simulink model "SimDraft2"  (R2024a)
settings: Solver=VariableStepAuto  StartTime=0.0  StopTime=2  RelTol=1e-3
model workspace (MAT data in the model file):
  CanaryAmplitude = 0
  CanaryCarrierFrequency = 20000
  CanaryDataRate = 100
  DataAmplitude = 1
  SampleRate = 44100
undefined symbols (not defined in the file or in its folder): magnitude
libraries: dspfdesign x3, audiosources x2, commseqgen3 x2, commchan3 x1, commanapbnd3 x1, phasedenvlib x1, commsync2 x1
settings Model: Creator=calum  LastModifiedBy=calum

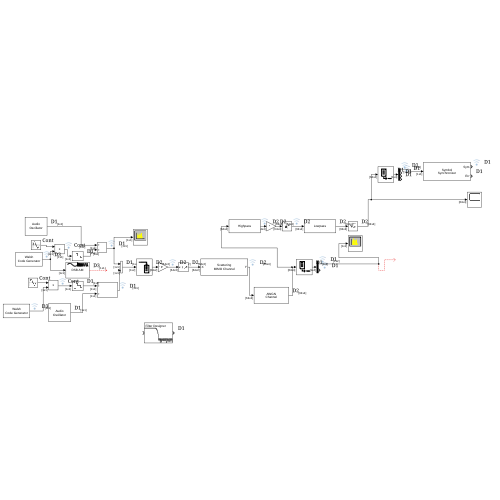
[thumbnail: Simulink's stored preview of the top-level diagram]
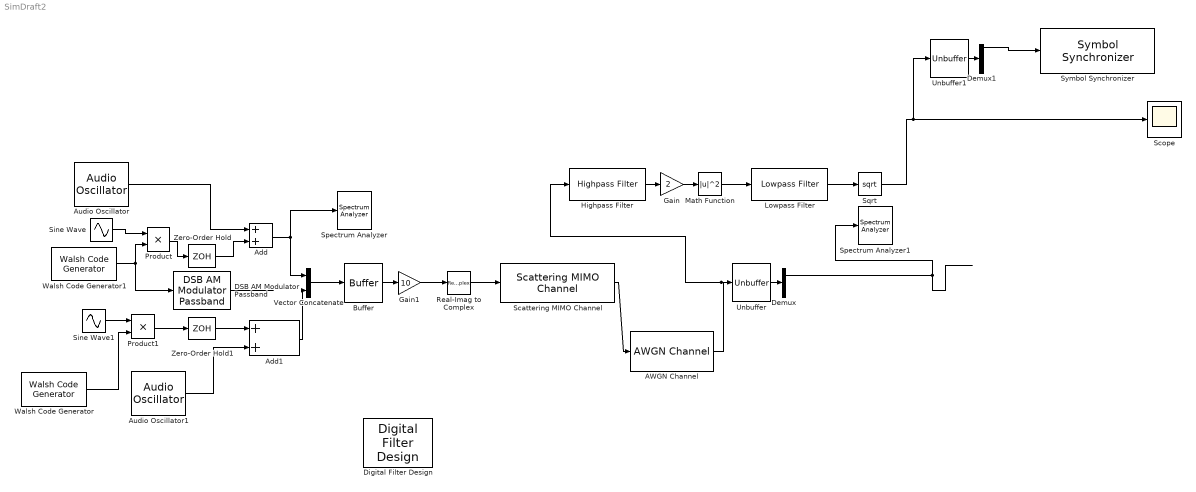
== system SimDraft2 ==
  AWGN Channel : commchan3/AWGN Channel  LegacyMode=off  NoiseMethod="Signal to noise ratio  (SNR)"  noiseMode="Signal to noise ratio  (SNR)"  EbNo=10  EsNo=10  SNR=70  BitsPerSymbol=1  SignalPower=1  SamplesPerSymbol=1  SymbolPeriod=1  VarianceSource=Parameter  Variance=1  RandomStream=Global stream  Seed=67  SimulateUsing=Code generation
  Add : Sum
  Add1 : Sum
  Audio Oscillator : audiosources/Audio Oscillator  FrequencyPort=off  Frequency=200  AmplitudePort=off  Amplitude=DataAmplitude  DCOffsetPort=off  DCOffset=0  PhaseOffset=0  WidthPort=off  Width=1  DutyCyclePort=off  DutyCycle=0.5  SampsPerFrame=1  Fs=SampleRate  OutputDataType=double  SimulateUsing=Code generation
      settings: SignalType=sine
  Audio Oscillator1 : audiosources/Audio Oscillator  FrequencyPort=off  Frequency=400  AmplitudePort=off  Amplitude=DataAmplitude  DCOffsetPort=off  DCOffset=0  PhaseOffset=0  WidthPort=off  Width=1  DutyCyclePort=off  DutyCycle=0.5  SampsPerFrame=1  Fs=SampleRate  OutputDataType=double  SimulateUsing=Code generation
      settings: SignalType=sine
  Buffer : Buffer  OutputFrames=off
  DSB AM Modulator Passband : commanapbnd3/DSB AM Modulator Passband  Fc=CanaryCarrierFrequency  Ph=0  Offset=1
  Demux : Demux  Outputs=2
  Demux1 : Demux
  Digital Filter Design : dspfdesign/Digital Filter Design  mwdsp_browser_bugfix_var=off
  Gain : Gain  Gain=2
  Gain1 : Gain  Gain=10
  Highpass Filter : dspfdesign/Highpass Filter  FilterType=FIR  DesignForMinimumOrder=on  FilterOrder=50  StopbandFrequency=CanaryCarrierFrequency-10*CanaryDataRate  PassbandFrequency=CanaryCarrierFrequency-4*CanaryDataRate  StopbandAttenuation=80  PassbandRipple=0.1  SampleRateMode=Specify on dialog  SampleRate=44100  SimulateUsing=Code generation  roundingMode=Floor  coeffsDataTypeStr=fixdt(1,16)
  Lowpass Filter : dspfdesign/Lowpass Filter  FilterType=FIR  DesignForMinimumOrder=on  FilterOrder=50  PassbandFrequency=CanaryDataRate  StopbandFrequency=CanaryDataRate*4  PassbandRipple=0.1  StopbandAttenuation=80  SampleRateMode=Specify on dialog  SampleRate=44100  SimulateUsing=Code generation  roundingMode=Floor  coeffsDataTypeStr=fixdt(1,16)
  Math Function : Math  Operator=magnitude^2
  Product : Product
  Product1 : Product
  Real-Imag to Complex : RealImagToComplex  Input=Real  ConstantPart=1E-3
  Scattering MIMO Channel : phasedenvlib/Scattering MIMO Channel  PropagationSpeed=300  CarrierFrequency=1  Polarization=None  SpecifyAtmosphere=off  Temperature=15  DryAirPressure=101325  WaterVapourDensity=7.5  LiquidWaterDensity=0  RainRate=0  SampleRateFromInputCheckbox=on  SampleRate=1e6  SimulateDirectPath=off  MaximumDelaySource=Property  MaximumDelay=2  ChannelResponseOutputPort=off  SimulateUsing=Code generation  TransmitArray=phased.ULA(Element=phased.OmnidirectionalMicrophoneElement(BackBaffled=false),ElementSpacing=20)  ReceiveArray=phased.ULA(Element=phased.OmnidirectionalMicrophoneElement(BackBaffled=false),ElementSpacing=10,NumElements=4)  TransmitArrayMotionSource=Property  TransmitArrayPosition=[ 0; 0; 0 ]  TransmitArrayOrientationAxes=eye( 3 )  ReceiveArrayMotionSource=Property  ReceiveArrayPosition=[ 1; 0; 0 ]  ReceiveArrayOrientationAxes=eye( 3 )  ScattererSpecificationSource=Property  NumScatterers=0  ScattererPositionBoundary=[ 0, 1000 ]  ScattererPosition=[ 0.5; 0; 0 ]  ScattererCoefficient=1  ScatteringMatrix=eye( 2 )  ScattererOrientationAxes=eye( 3 )  SeedSource=Auto  Seed=0
  Scope : Scope
  Sine Wave : Sin  Amplitude=CanaryAmplitude  Frequency=2*pi*CanaryCarrierFrequency  SampleTime=0
  Sine Wave1 : Sin  Amplitude=CanaryAmplitude  Frequency=2*pi*CanaryCarrierFrequency  SampleTime=0
  Spectrum Analyzer : SpectrumAnalyzer  WindowPosition=[713.000000,244.000000,800.000000,500.000000,]  Visible=on  ScopeFrameLocation=window  SampleRateSource=Property  SampleRate=44.1e3  PlotAsTwoSidedSpectrum=off  FrequencyScale=Log  FrequencySpan=Start and stop frequencies  StartFrequency=20  StopFrequency=20e3  YLimits=[-63.59812407,36.96716978]
  Spectrum Analyzer1 : SpectrumAnalyzer  WindowPosition=[314.000000,172.000000,1126.000000,498.000000,]  Visible=on  ScopeFrameLocation=window  SampleRateSource=Property  SampleRate=44.1e3  PlotAsTwoSidedSpectrum=off  FrequencyScale=Log  FrequencySpan=Start and stop frequencies  StartFrequency=20  StopFrequency=20e3  YLimits=[-37.37791181,56.27526663]
  Sqrt : Sqrt
  Symbol Synchronizer : commsync2/Symbol Synchronizer  Modulation=PAM/PSK/QAM  TimingErrorDetector=Zero-Crossing (decision-directed)  SamplesPerSymbol=SampleRate/CanaryDataRate*2  DampingFactor=1  NormalizedLoopBandwidth=0.01  DetectorGain=2.7  TimingErrorOutputPort=on  SimulateUsing=Code generation
  Unbuffer : Unbuffer
  Unbuffer1 : Unbuffer
  Vector Concatenate : Concatenate  Mode=Multidimensional array  ConcatenateDimension=2
  Walsh Code Generator : commseqgen3/Walsh Code Generator  Length=16  Index=8  SampleTime=1/CanaryDataRate  SamplesPerFrame=1  OutputDataType=double  SimulateUsing=Code generation
  Walsh Code Generator1 : commseqgen3/Walsh Code Generator  Length=16  Index=8  SampleTime=1/CanaryDataRate  SamplesPerFrame=1  OutputDataType=double  SimulateUsing=Code generation
  Zero-Order Hold : ZeroOrderHold  SampleTime=1/SampleRate
  Zero-Order Hold1 : ZeroOrderHold  SampleTime=1/SampleRate
  wires:
  Vector Concatenate/1 -> Buffer/1
  Sine Wave/1 -> Product/1
  Sine Wave1/1 -> Product1/1
  Walsh Code Generator/1 -> Product1/2
  Product/1 -> Zero-Order Hold/1
  Audio Oscillator/1 -> Add/1
  Add/1 -> Vector Concatenate/1, Spectrum Analyzer/1
  Add1/1 -> Vector Concatenate/2
  Product1/1 -> Zero-Order Hold1/1
  Audio Oscillator1/1 -> Add1/2
  Scattering MIMO Channel/1 -> AWGN Channel/1
  Zero-Order Hold/1 -> Add/2
  Zero-Order Hold1/1 -> Add1/1
  Buffer/1 -> Gain1/1
  Unbuffer/1 -> Demux/1
  Demux/1 -> Spectrum Analyzer1/1
  DSB AM Modulator Passband/1 -> ?
  Walsh Code Generator1/1 -> Product/2, DSB AM Modulator Passband/1
  AWGN Channel/1 -> Highpass Filter/1, Unbuffer/1
  Math Function/1 -> Lowpass Filter/1
  Lowpass Filter/1 -> Sqrt/1
  Gain/1 -> Math Function/1
  Sqrt/1 -> Unbuffer1/1, Scope/1
  Unbuffer1/1 -> Demux1/1
  Demux1/1 -> Symbol Synchronizer/1
  Highpass Filter/1 -> Gain/1
  Gain1/1 -> Real-Imag to Complex/1
  Real-Imag to Complex/1 -> Scattering MIMO Channel/1
